simulink model "lab1_bd"  (R2021a)
settings: Solver=VariableStepAuto  StartTime=0.0  StopTime=8  RelTol=1e-3
libraries: simulink x3
settings Model: Creator=LEGION  LastModifiedBy=LEGION

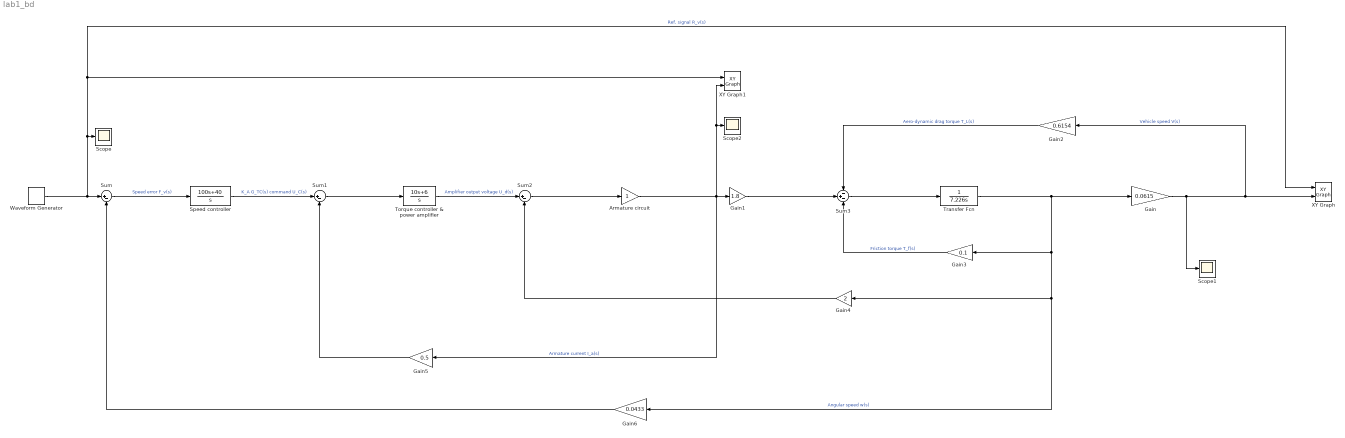
== system lab1_bd ==
  Armature circuit : Gain
  Gain : Gain  Gain=0.0615
  Gain1 : Gain  Gain=1.8
  Gain2 : Gain  Gain=0.6154
  Gain3 : Gain  Gain=0.1
  Gain4 : Gain  Gain=2
  Gain5 : Gain  Gain=0.5
  Gain6 : Gain  Gain=0.0433
  Scope : Scope
  Scope1 : Scope
  Scope2 : Scope
  Speed controller : TransferFcn  Numerator=[100 40]  Denominator=[1 0]  ContinuousStateAttributes='speed_controller'
  Sum : Sum  Inputs=|+-
  Sum1 : Sum  Inputs=|+-
  Sum2 : Sum  Inputs=|+-
  Sum3 : Sum  Inputs=-+-
  Torque controller & power amplifier : TransferFcn  Numerator=[10 6]  Denominator=[1 0]  ContinuousStateAttributes='torque_controller'
  Transfer Fcn : TransferFcn  Denominator=[7.226 0]  ContinuousStateAttributes='motor_inertia'
  Waveform Generator : simulink/Sources/Waveform Generator  OutMin=[]  OutMax=[]  OutDataTypeStr=double  SelectedSignal=3  Signals=square('Amplitude',5,'Frequency',5,'Phase',0,'DutyCycle',80)#square('Amplitude',5,'Frequency',2*pi*5,'Phase',0,'DutyCycle',80)#square('Amplitude',5,'Frequency',31.4159,'Phase',0,'DutyCycle',80)  BlockNames=MultiportSwitch_99bb250074db4f6#MultiportSwitch_12e6e47c333f4b2#MultiportSwitch_c2328080b0a34ab  SampleTime=0.01
  XY Graph : simulink/Sinks/XY Graph  xmin=-inf  xmax=inf  ymin=-inf  ymax=inf  st=0.01
  XY Graph1 : simulink/Sinks/XY Graph  xmin=-inf  xmax=inf  ymin=-inf  ymax=inf  st=0.01
  wires:
  Waveform Generator/1 -> XY Graph1/1, XY Graph/1, Scope/1, Sum/1  "Ref. signal R_v(s)"
  Sum/1 -> Speed controller/1  "Speed error F_v(s)"
  Speed controller/1 -> Sum1/1  "K_A G_TC(s) command U_C(s)"
  Sum1/1 -> Torque controller & power amplifier/1
  Torque controller & power amplifier/1 -> Sum2/1  "Amplifier output voltage U_d(s)"
  Sum2/1 -> Armature circuit/1
  Armature circuit/1 -> XY Graph1/2, Scope2/1, Gain5/1, Gain1/1  "Armature current I_a(s)"
  Gain1/1 -> Sum3/2
  Sum3/1 -> Transfer Fcn/1
  Transfer Fcn/1 -> Gain6/1, Gain4/1, Gain3/1, Gain/1  "Angular speed w(s)"
  Gain2/1 -> Sum3/1  "Aero-dynamic drag torque T_L(s)"
  Gain3/1 -> Sum3/3  "Friction torque T_f(s)"
  Gain4/1 -> Sum2/2
  Gain5/1 -> Sum1/2
  Gain6/1 -> Sum/2
  Gain/1 -> Scope1/1, XY Graph/2, Gain2/1  "Vehicle speed V(s)"
